simulink model "adaptive_ctrl_2021_05_01"  (R2020a)
settings: Solver=VariableStepAuto  StartTime=0.0  StopTime=simlength  MaxStep=Tc  RelTol=1e-3
values from neighbouring files (symbols this model uses):
  A = [0 1; 0 0]    [init_adaptive.m]
  a_ref = 1    [init_adaptive.m]
  Am = [0 1; -lambda2 -lambda1]    [init_adaptive.m]
  B = [0 1/m]'    [init_adaptive.m]
  Bm = [0 lambda2]'    [init_adaptive.m]
  C = [1 0]    [init_adaptive.m]
  Cm = [1 0]    [init_adaptive.m]
  gamma = 0.5    [init_adaptive.m]
  L = acker(Aobs',Cobs',[-50, -100])    [init_adaptive.m]
  lambda = 6    [init_adaptive.m]
  m = 2    [init_adaptive.m]
  Tc = 1e-5    (= 1e-05)    [init_adaptive.m]
  w_ref = 4    [init_adaptive.m]
settings Model: Creator=dbagn  LastModifiedBy=dbagn
settings DataIOCC: ReturnWorkspaceOutputs=off
settings SFSimCC: CustomCodeUndefinedFunction=UseInterfaceOnly

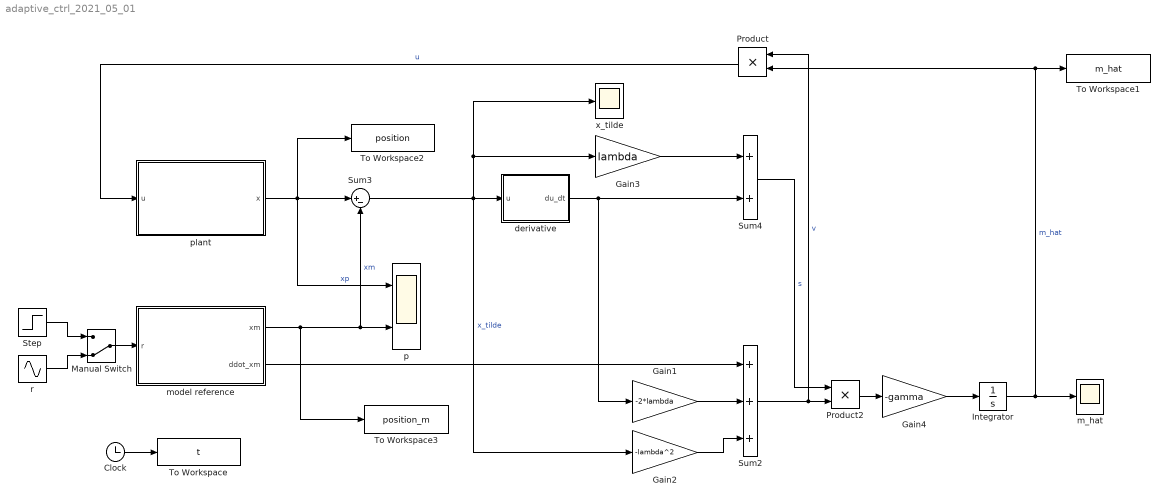
== system adaptive_ctrl_2021_05_01 ==
  Clock : Clock
  Gain1 : Gain  Gain=-2*lambda
  Gain2 : Gain  Gain=-lambda^2
  Gain3 : Gain  Gain=lambda
  Gain4 : Gain  Gain=-gamma
  Integrator : Integrator  InitialCondition=0 %m*0.85
  Manual Switch : ManualSwitch  CurrentSetting=0
  Product : Product
  Product2 : Product
  Step : Step  Time=0.2  After=2  SampleTime=0
  Sum2 : Sum  Inputs=+++
  Sum3 : Sum  Inputs=|+-
  Sum4 : Sum
  To Workspace : ToWorkspace  VariableName=t  SampleTime=Tc
      settings: MaxDataPoints=Nc
  To Workspace1 : ToWorkspace  VariableName=m_hat  SampleTime=Tc
      settings: MaxDataPoints=Nc
  To Workspace2 : ToWorkspace  VariableName=position  SampleTime=Tc
      settings: MaxDataPoints=Nc
  To Workspace3 : ToWorkspace  VariableName=position_m  SampleTime=Tc
      settings: MaxDataPoints=Nc
  derivative : Subsystem
  m_hat : Scope
  model reference : Subsystem
  p : Scope  NumInputPorts=2
  "plant " : Subsystem
  r : Sin  Amplitude=a_ref  Frequency=w_ref  SampleTime=0
  x_tilde : Scope
  wires:
  "plant "/1(x) -> Sum3/1, p/1, To Workspace2/1  "xp"
  model reference/1(xm) -> To Workspace3/1, p/2, Sum3/2  "xm"
  Sum3/1 -> x_tilde/1, Gain3/1, Gain2/1, derivative/1(u)  "x_tilde"
  Product/1 -> "plant "/1(u)  "u"
  model reference/2(ddot_xm) -> Sum2/1
  Gain1/1 -> Sum2/2
  Gain2/1 -> Sum2/3
  derivative/1(du_dt) -> Gain1/1, Sum4/2
  Sum2/1 -> Product2/2, Product/1  "v"
  Gain3/1 -> Sum4/1
  Sum4/1 -> Product2/1  "s"
  Product2/1 -> Gain4/1
  Gain4/1 -> Integrator/1
  Integrator/1 -> To Workspace1/1, Product/2, m_hat/1  "m_hat"
  Clock/1 -> To Workspace/1
  Manual Switch/1 -> model reference/1(r)
  r/1 -> Manual Switch/2
  Step/1 -> Manual Switch/1

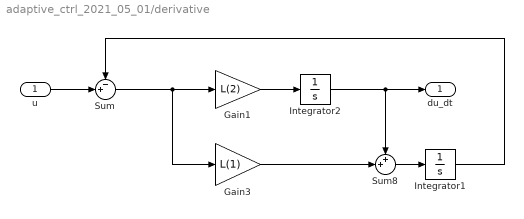
== system adaptive_ctrl_2021_05_01/derivative ==
  u : Inport
  Gain1 : Gain  Gain=L(2)
  Gain3 : Gain  Gain=L(1)
  Integrator1 : Integrator
  Integrator2 : Integrator
  Sum : Sum  Inputs=-+|
  Sum8 : Sum  Inputs=++|
  du_dt : Outport  VectorParamsAs1DForOutWhenUnconnected=off
  wires:
  Sum8/1 -> Integrator1/1
  u/1 -> Sum/2
  Integrator1/1 -> Sum/1
  Gain1/1 -> Integrator2/1
  Sum/1 -> Gain3/1, Gain1/1
  Gain3/1 -> Sum8/2
  Integrator2/1 -> du_dt/1, Sum8/1

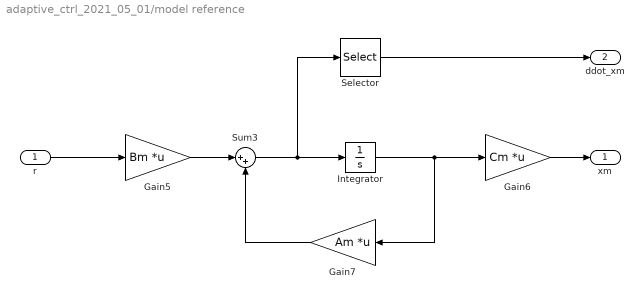
== system adaptive_ctrl_2021_05_01/model reference ==
  r : Inport
  Gain5 : Gain  Gain=Bm  Multiplication=Matrix(K*u)
  Gain6 : Gain  Gain=Cm  Multiplication=Matrix(K*u)
  Gain7 : Gain  Gain=Am  Multiplication=Matrix(K*u)
  Integrator : Integrator
  Selector : Selector  InputPortWidth=2  IndexOptions=Index vector (dialog)  Indices=2  OutputSizes=1
  Sum3 : Sum  Inputs=|++
  xm : Outport
  ddot_xm : Outport  Port=2
  wires:
  Integrator/1 -> Gain6/1, Gain7/1
  Gain6/1 -> xm/1
  Gain5/1 -> Sum3/1
  r/1 -> Gain5/1
  Gain7/1 -> Sum3/2
  Sum3/1 -> Selector/1, Integrator/1
  Selector/1 -> ddot_xm/1

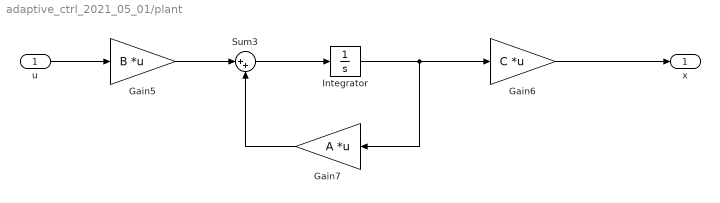
== system adaptive_ctrl_2021_05_01/plant  ==
  u : Inport
  Gain5 : Gain  Gain=B  Multiplication=Matrix(K*u)
  Gain6 : Gain  Gain=C  Multiplication=Matrix(K*u)
  Gain7 : Gain  Gain=A  Multiplication=Matrix(K*u)
  Integrator : Integrator
  Sum3 : Sum  Inputs=|++
  x : Outport
  wires:
  Sum3/1 -> Integrator/1
  Gain7/1 -> Sum3/2
  u/1 -> Gain5/1
  Gain5/1 -> Sum3/1
  Gain6/1 -> x/1
  Integrator/1 -> Gain7/1, Gain6/1
